simulink model "Assignment_II_extraB"  (R2024b)
settings: Solver=FixedStepAuto  StartTime=0.0  StopTime=inf  FixedStep=1/f_cmd  RelTol=1e-3
values from neighbouring files (symbols this model uses):
  ang_max = 0.05    [Assignment_II.m]
  dist_max = 0.01    [Assignment_II.m]
  k1 = 3    [Assignment_II.m]
  k2 = 5    [Assignment_II.m]
  k3 = 4    [Assignment_II.m]
  turtlebot3 = [ ... (first row only)    [Assignment_II.m]
  v_max = 0.2    [Assignment_II.m]
  yaw_rate_max = 0.4    [Assignment_II.m]
undefined symbols (not defined in the file or in its folder): Angular, Linear
libraries: robotlib x3, simulink x1
settings Model: PacingRate=20  Creator=vigno  LastModifiedBy=vigno
settings OptimizationCC: EnhancedBackFolding=on  PassReuseOutputArgsAs=Individual arguments  ZeroExternalMemoryAtStartup=off  ZeroInternalMemoryAtStartup=off  MaxStackSize=64  OptimizeBlockOrder=speed  DifferentSizesBufferReuse=on  OptimizationCustomize=off  EfficientTunableParamExpr=on
settings DebuggingCC: ParameterTunabilityLossMsg=error
settings HardwareCC: ProdBitPerPointer=32  ProdBitPerSizeT=32  ProdBitPerPtrDiffT=32  ProdLargestAtomicFloat=None  ProdIntDivRoundTo=Undefined  ProdEndianess=Unspecified  ProdWordSize=32  ProdHWDeviceType=Generic->Unspecified (assume 32-bit Generic)
settings ModelReferenceCC: EnableRefExpFcnMdlSchedulingChecks=on
settings SFSimCC: MATLABDynamicMemAlloc=off
settings RTWCC: Description=Embedded Coder  SystemTargetFile=ert.tlc  HardwareBoard=Robot Operating System (ROS)  TLCOptions="-aInlineSetEventsForThisBaseRateFcn=TLC_FALSE -aSuppressMultiTaskScheduler=TLC_FALSE  -aRateBasedStepFcn=0"  TemplateMakefile=ert_default_tmf  Toolchain=Catkin  TargetLang=C++  GPUComputeCapability=3.5
settings CodeAppCC: ForceParamTrailComments=on  IgnoreCustomStorageClasses=off  OperatorAnnotations=on  SimulinkDataObjDesc=on  SFDataObjDesc=on  InsertBlockDesc=on
settings ERTTargetCC: InlinedParameterPlacement=Hierarchical  DynamicArrayContainerType=coder::array

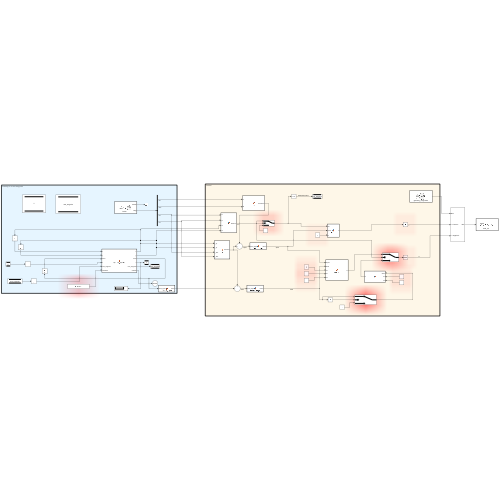
[thumbnail: Simulink's stored preview of the top-level diagram]
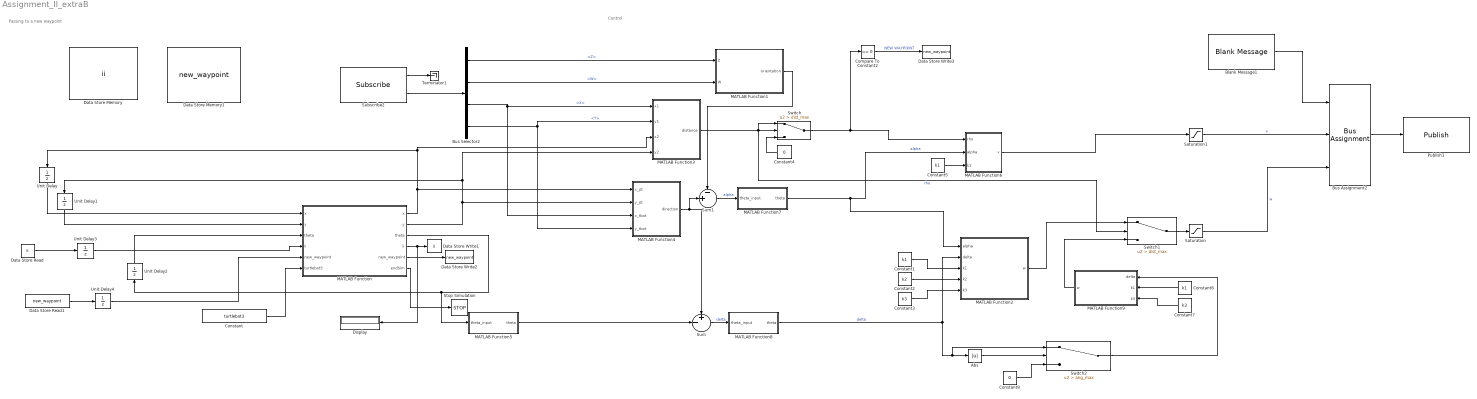
== system Assignment_II_extraB ==
  note: Passing to a new waypoint
  note: Control
  Abs : Abs  SaturateOnIntegerOverflow=off
  Blank Message1 : robotlib/Blank Message  messageClass=Message  entityType=geometry_msgs/Twist  messageType=geometry_msgs/Twist  SampleTime=-1  legacyBusStruct=off
  Bus Assignment2 : BusAssignment  AssignedSignals=Linear.X,Angular.Z
  Bus Selector2 : BusSelector  OutputSignals=Pose.Pose.Orientation.Z,Pose.Pose.Orientation.W,Pose.Pose.Position.X,Pose.Pose.Position.Y
  Compare To Constant2 : simulink/Logic and Bit Operations/Compare To Constant  relop===  const=0  OutDataTypeStr=boolean
  Constant : Constant  Value=turtlebot3
  Constant1 : Constant  Value=k1
  Constant2 : Constant  Value=k2
  Constant3 : Constant  Value=k3
  Constant4 : Constant  Value=0
  Constant5 : Constant  Value=k1
  Constant6 : Constant  Value=k1
  Constant7 : Constant  Value=k3
  Constant8 : Constant  Value=0
  Data Store Memory : DataStoreMemory  DataStoreName=ii  WriteAfterWriteMsg=warning  ShowAdditionalParam=off  OutDataTypeStr=double
  Data Store Memory1 : DataStoreMemory  DataStoreName=new_waypoint  WriteAfterWriteMsg=warning  ShowAdditionalParam=off
  Data Store Read : DataStoreRead  DataStoreName=ii  DataStoreElements=ii  IndexOptions=Index vector (dialog)  Indices=1  OutputSizes=1
  Data Store Read1 : DataStoreRead  DataStoreName=new_waypoint  DataStoreElements=new_waypoint  IndexOptions=Index vector (dialog)  Indices=1  OutputSizes=1
  Data Store Write1 : DataStoreWrite  DataStoreName=ii  DataStoreElements=ii  IndexOptions=Index vector (dialog)  Indices=1  OutputSizes=1
  Data Store Write2 : DataStoreWrite  DataStoreName=new_waypoint  DataStoreElements=new_waypoint  IndexOptions=Index vector (dialog)  Indices=1  OutputSizes=1
  Data Store Write3 : DataStoreWrite  DataStoreName=new_waypoint  IndexOptions=Index vector (dialog)  Indices=1  OutputSizes=1
  Display : Display
  MATLAB Function : MATLAB Function  TreatAsAtomicUnit=on
  MATLAB Function1 : MATLAB Function  TreatAsAtomicUnit=on
  MATLAB Function2 : MATLAB Function  TreatAsAtomicUnit=on
  MATLAB Function3 : MATLAB Function  TreatAsAtomicUnit=on
  MATLAB Function4 : MATLAB Function  TreatAsAtomicUnit=on
  MATLAB Function5 : MATLAB Function  TreatAsAtomicUnit=on
  MATLAB Function6 : MATLAB Function  TreatAsAtomicUnit=on
  MATLAB Function7 : MATLAB Function  TreatAsAtomicUnit=on
  MATLAB Function8 : MATLAB Function  TreatAsAtomicUnit=on
  MATLAB Function9 : MATLAB Function  TreatAsAtomicUnit=on
  Publish1 : robotlib/Publish  topicSource=Select from ROS network  topic=/cmd_vel  messageType=geometry_msgs/Twist  legacyBusStruct=off  messageQueueLength=1
  Saturation : Saturate  UpperLimit=yaw_rate_max  LowerLimit=- yaw_rate_max
  Saturation1 : Saturate  UpperLimit=v_max  LowerLimit=- v_max
  Stop Simulation : Stop
  Subscribe2 : robotlib/Subscribe  topicSource=Select from ROS network  topic=/odom  messageType=nav_msgs/Odometry  SampleTime=-1  legacyBusStruct=off  messageQueueLength=1
  Sum : Sum  Inputs=+-|
  Sum1 : Sum  Inputs=-+|
  Switch : Switch  Criteria=u2 > Threshold  Threshold=dist_max  SaturateOnIntegerOverflow=off  InputSameDT=off
  Switch1 : Switch  Criteria=u2 > Threshold  Threshold=dist_max  SaturateOnIntegerOverflow=off  InputSameDT=off
  Switch2 : Switch  Criteria=u2 > Threshold  Threshold=ang_max  SaturateOnIntegerOverflow=off  InputSameDT=off
  Terminator1 : Terminator
  Unit Delay{,1..4} (5 alike) : UnitDelay  SampleTime=-1  HasFrameUpgradeWarning=on
  wires:
  Subscribe2/2 -> Bus Selector2/1
  Blank Message1/1 -> Bus Assignment2/1
  Bus Selector2/2 -> MATLAB Function1/2(W)  "<W>"
  Bus Assignment2/1 -> Publish1/1
  Subscribe2/1 -> Terminator1/1
  Bus Selector2/4 -> MATLAB Function3/2(y1), MATLAB Function4/4(y_tbot)  "<Y>"
  Bus Selector2/1 -> MATLAB Function1/1(Z)  "<Z>"
  Bus Selector2/3 -> MATLAB Function4/3(x_tbot), MATLAB Function3/1(x1)  "<X>"
  Compare To Constant2/1 -> Data Store Write3/1  "NEW WAYPOINT"
  Data Store Read/1 -> Unit Delay3/1
  Data Store Read1/1 -> Unit Delay4/1
  MATLAB Function/2(y) -> MATLAB Function4/2(y_pt), MATLAB Function3/4(y2), Unit Delay1/1
  MATLAB Function/1(x) -> MATLAB Function4/1(x_pt), MATLAB Function3/3(x2), Unit Delay/1
  MATLAB Function/4(ii) -> Display/1, Data Store Write1/1
  MATLAB Function/5(new_waypoint) -> Data Store Write2/1
  MATLAB Function/6(endSim) -> Stop Simulation/1
  Constant/1 -> MATLAB Function/6(turtlebot3)
  Unit Delay/1 -> MATLAB Function/1("x ")
  Unit Delay1/1 -> MATLAB Function/2("y ")
  Unit Delay2/1 -> MATLAB Function/3("theta ")
  Unit Delay3/1 -> MATLAB Function/4("ii ")
  Unit Delay4/1 -> MATLAB Function/5("new_waypoint ")
  Saturation/1 -> Bus Assignment2/3  "w"
  MATLAB Function/3(theta) -> MATLAB Function5/1(theta_input), Unit Delay2/1
  Saturation1/1 -> Bus Assignment2/2  "v"
  MATLAB Function5/1(theta) -> Sum/2
  MATLAB Function4/1(direction) -> Sum/1, Sum1/2
  MATLAB Function1/1(orientation) -> Sum1/1
  Constant1/1 -> MATLAB Function2/3(k1)
  Constant2/1 -> MATLAB Function2/4(k2)
  Constant3/1 -> MATLAB Function2/5(k3)
  MATLAB Function3/1(distance) -> Switch1/2, Switch/1, Switch/2  "rho"
  Constant4/1 -> Switch/3
  Sum/1 -> MATLAB Function8/1(theta_input)  "delta"
  Sum1/1 -> MATLAB Function7/1(theta_input)  "alpha"
  Switch/1 -> Compare To Constant2/1, MATLAB Function6/1(rho)
  Constant5/1 -> MATLAB Function6/3(k1)
  MATLAB Function7/1(theta) -> MATLAB Function2/1(alpha), MATLAB Function6/2(alpha)  "alpha"
  MATLAB Function8/1(theta) -> MATLAB Function2/2(delta), Switch2/1, Abs/1  "delta"
  MATLAB Function6/1(v) -> Saturation1/1
  MATLAB Function2/1(w) -> Switch1/1
  MATLAB Function9/1(w) -> Switch1/3
  Constant6/1 -> MATLAB Function9/2(k1)
  Constant7/1 -> MATLAB Function9/3(k3)
  Abs/1 -> Switch2/2
  Constant8/1 -> Switch2/3
  Switch2/1 -> MATLAB Function9/1(delta)
  Switch1/1 -> Saturation/1

== matlab function Assignment_II_extraB/MATLAB Function8 ==
  data: theta_input input; theta output
function theta = correct_angle(theta_input)
    if theta_input <= pi && theta_input >= -pi
        theta = theta_input;
    else
        theta = mod(theta_input + pi, 2 * pi) - pi;
    end
end

== matlab function Assignment_II_extraB/MATLAB Function9 ==
  data: delta input; w output; k1 input; k3 input
function w = omega_close(delta, k1, k3)
    w = k1*k3*delta;
end

== matlab function Assignment_II_extraB/MATLAB Function2 ==
  data: alpha input; w output; delta input; k1 input; k2 input; k3 input
function w = omega(alpha, delta, k1, k2, k3)

    w = k2*alpha + k1*sin(alpha)*cos(alpha)/(alpha + 1e-5) * (alpha + k3*delta);

end

== matlab function Assignment_II_extraB/MATLAB Function ==
  data: x input; y input; theta input; ii input; x output; y output; new_waypoint input; theta output; ii output; new_waypoint output; turtlebot3 input; endSim output
function [x, y, theta, ii, new_waypoint, endSim] = new_waypointer(x, y, theta, ii, new_waypoint, turtlebot3)
    endSim = false;
    if new_waypoint
        ii = double(ii);
        ii = ii + 1;
        if ii > size(turtlebot3, 1)
            endSim = true;
            return
        else
            x = turtlebot3(ii, 1);
            y = turtlebot3(ii, 2);
            theta = turtlebot3(ii, 3);
        end
    end
end

== matlab function Assignment_II_extraB/MATLAB Function5 ==
  data: theta_input input; theta output
function theta = correct_angle(theta_input)
    if theta_input <= pi && theta_input >= -pi
        theta = theta_input;
    else
        theta = mod(theta_input + pi, 2 * pi) - pi;
    end
end

== matlab function Assignment_II_extraB/MATLAB Function6 ==
  data: rho input; v output; alpha input; k1 input
function v = speed(rho, alpha, k1)

    v = k1 * rho * cos(alpha);

end

== matlab function Assignment_II_extraB/MATLAB Function1 ==
  data: Z input; orientation output; W input
function orientation = fcn(Z, W)
    orientation = 2 * atan2(Z, W);
    if orientation > pi
        orientation = orientation - 2 * pi;
    elseif orientation < -pi
        orientation = orientation + 2 * pi;
    end
end

== matlab function Assignment_II_extraB/MATLAB Function3 ==
  data: x1 input; distance output; y1 input; x2 input; y2 input
function distance = fcn(x1, y1, x2, y2)
    distance = sqrt((x1 - x2)^2 + (y1 - y2)^2);

== matlab function Assignment_II_extraB/MATLAB Function4 ==
  data: x_pt input; direction output; y_pt input; x_tbot input; y_tbot input
function direction = fcn(x_pt, y_pt, x_tbot, y_tbot)
    direction = atan2(y_pt - y_tbot, x_pt - x_tbot);

== matlab function Assignment_II_extraB/MATLAB Function7 ==
  data: theta_input input; theta output
function theta = correct_angle(theta_input)
    if theta_input <= pi && theta_input >= -pi
        theta = theta_input;
    else
        theta = mod(theta_input + pi, 2 * pi) - pi;
    end
end
